simulink model "lab3m2"  (R2018a)
settings: Solver=ode4  StartTime=0.0  StopTime=10.0  FixedStep=1e-2  RelTol=1e-3
values from neighbouring files (symbols this model uses):
  A = [0,1;-6,-5]    [MarcinGrzybSkrypt.m]
  Apl = expm(stime*A)    [MarcinGrzybSkrypt.m]
  B = [0;1]    [MarcinGrzybSkrypt.m]
  Bpl = double(int(expm(x*A)*B,x,0,stime))    [MarcinGrzybSkrypt.m]
  C = [1,0;0,1]    [MarcinGrzybSkrypt.m]
  Cpl = C    [MarcinGrzybSkrypt.m]
  D = [0;0]    [MarcinGrzybSkrypt.m]
  stime = 0.1    [MarcinGrzybSkrypt.m]
  WPC = 0.5    [MarcinGrzybSkrypt.m]
settings Model: Creator=nicra  LastModifiedBy=nicra

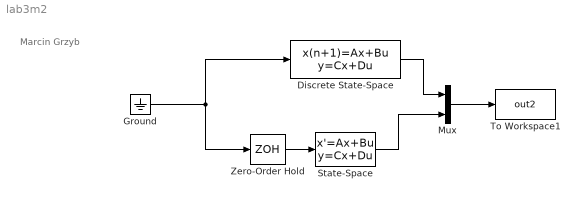
== system lab3m2 ==
  note: Marcin Grzyb
  Discrete State-Space : DiscreteStateSpace  A=Apl  B=Bpl  C=Cpl  D=[0;0]  InitialCondition=WPC  SampleTime=stime
  Ground : Ground
  Mux : Mux  Inputs=2
  State-Space : StateSpace  A=A  B=B  C=C  D=D  InitialCondition=WPC
  To Workspace1 : ToWorkspace  VariableName=out2  SampleTime=-1
  Zero-Order Hold : ZeroOrderHold  SampleTime=stime
  wires:
  Discrete State-Space/1 -> Mux/1
  State-Space/1 -> Mux/2
  Mux/1 -> To Workspace1/1
  Zero-Order Hold/1 -> State-Space/1
  Ground/1 -> Discrete State-Space/1, Zero-Order Hold/1
